simulink model "singlcontact_control_smc_lqr_mydimes_reaction"  (R2024a)
settings: Solver=VariableStepAuto  StartTime=0.0  StopTime=10  FixedStep=0.001  RelTol=1e-3
values from neighbouring files (symbols this model uses):
  ankle_servo_kd = 8    [robotParametersCtrl_mydiem_block_zmp.m]    (also in robotParametersCtrl_quad_modify_mydiem.m; robotParametersCtrl_quad_modify_mydiem_reaction.m)
  ankle_servo_ki = 4    [robotParametersCtrl_mydiem_block_zmp.m]    (also in robotParametersCtrl_quad_modify_mydiem.m; robotParametersCtrl_quad_modify_mydiem_reaction.m)
  ankle_servo_kp = 20    [robotParametersCtrl_mydiem_block_zmp.m]    (also in robotParametersCtrl_quad_modify_mydiem.m; robotParametersCtrl_quad_modify_mydiem_reaction.m)
  deriv_filter_coeff = 100    [robotParametersCtrl_mydiem_block_zmp.m]    (also in robotParametersCtrl_quad_modify_mydiem.m; robotParametersCtrl_quad_modify_mydiem_reaction.m)
  filter_coefficent_pid = 100    [robotParametersCtrl_mydiem_block_zmp.m]    (also in robotParametersCtrl_quad_modify_mydiem.m; robotParametersCtrl_quad_modify_mydiem_reaction.m)
  filter_coefficent_pids = 100    [robotParametersCtrl_quad_modify_mydiem_reaction.m]
  foot_z = 1.5    [robotParametersCtrl_mydiem_block_zmp.m]    (also in robotParametersCtrl_quad_modify_mydiem.m; robotParametersCtrl_quad_modify_mydiem_reaction.m)
  g = 9.81    [ABCDvalues_lqr_quad_mydime_reaction.m]    (also in robotParametersCtrl_mydiem_block_zmp.m = 9.80665; robotParametersCtrl_quad_modify_mydiem.m = 9.80665; robotParametersCtrl_quad_modify_mydiem_reaction.m = 9.80665)
  h = 32    [robotParametersCtrl_mydiem_block_zmp.m]    (also in robotParametersCtrl_quad_modify_mydiem.m; robotParametersCtrl_quad_modify_mydiem_reaction.m)
  height_plane = 0.025    [robotParametersCtrl_mydiem_block_zmp.m]    (also in robotParametersCtrl_quad_modify_mydiem.m; robotParametersCtrl_quad_modify_mydiem_reaction.m)
  hip_pitch_deriv = 20    [robotParametersCtrl_mydiem_block_zmp.m]    (also in robotParametersCtrl_quad_modify_mydiem.m = 200; robotParametersCtrl_quad_modify_mydiem_reaction.m = 200)
  hip_pitch_derivs = 200    [robotParametersCtrl_quad_modify_mydiem_reaction.m]
  hip_pitch_int = 0    [robotParametersCtrl_mydiem_block_zmp.m]    (also in robotParametersCtrl_quad_modify_mydiem.m = 150; robotParametersCtrl_quad_modify_mydiem_reaction.m = 150)
  hip_pitch_ints = 1500    [robotParametersCtrl_quad_modify_mydiem_reaction.m]
  hip_pitch_prop = 10    [robotParametersCtrl_mydiem_block_zmp.m]    (also in robotParametersCtrl_quad_modify_mydiem.m = 500; robotParametersCtrl_quad_modify_mydiem_reaction.m = 500)
  hip_pitch_props = 500    [robotParametersCtrl_quad_modify_mydiem_reaction.m]
  hip_roll_deriv = 28    [robotParametersCtrl_mydiem_block_zmp.m]    (also in robotParametersCtrl_quad_modify_mydiem.m = 280; robotParametersCtrl_quad_modify_mydiem_reaction.m = 280)
  hip_roll_derivs = 280    [robotParametersCtrl_quad_modify_mydiem_reaction.m]
  hip_roll_int = 0    [robotParametersCtrl_mydiem_block_zmp.m]    (also in robotParametersCtrl_quad_modify_mydiem.m = 180; robotParametersCtrl_quad_modify_mydiem_reaction.m = 180)
  hip_roll_ints = 180    [robotParametersCtrl_quad_modify_mydiem_reaction.m]
  hip_roll_prop = 10    [robotParametersCtrl_mydiem_block_zmp.m]    (also in robotParametersCtrl_quad_modify_mydiem.m = 300; robotParametersCtrl_quad_modify_mydiem_reaction.m = 300)
  hip_roll_props = 300    [robotParametersCtrl_quad_modify_mydiem_reaction.m]
  hip_servo_kd = 20    [robotParametersCtrl_mydiem_block_zmp.m]    (also in robotParametersCtrl_quad_modify_mydiem.m; robotParametersCtrl_quad_modify_mydiem_reaction.m)
  hip_servo_ki = 10    [robotParametersCtrl_mydiem_block_zmp.m]    (also in robotParametersCtrl_quad_modify_mydiem.m; robotParametersCtrl_quad_modify_mydiem_reaction.m)
  hip_servo_kp = 60    [robotParametersCtrl_mydiem_block_zmp.m]    (also in robotParametersCtrl_quad_modify_mydiem.m; robotParametersCtrl_quad_modify_mydiem_reaction.m)
  hip_smc_lamda = 85    [robotParametersCtrl_mydiem_block_zmp.m]    (also in robotParametersCtrl_quad_modify_mydiem.m; robotParametersCtrl_quad_modify_mydiem_reaction.m = 95)
  hip_smc_lamdas = 85    [robotParametersCtrl_quad_modify_mydiem_reaction.m]
  hip_smc_new = 25    [robotParametersCtrl_mydiem_block_zmp.m]    (also in robotParametersCtrl_quad_modify_mydiem.m; robotParametersCtrl_quad_modify_mydiem_reaction.m = 45)
  hip_smc_news = 25    [robotParametersCtrl_quad_modify_mydiem_reaction.m]
  init_angs_L = init_angs_R    [robotParametersCtrl_mydiem_block_zmp.m]    (also in robotParametersCtrl_quad_modify_mydiem.m; robotParametersCtrl_quad_modify_mydiem_reaction.m)
  init_angs_R = [0 -sum(init_angs) init_angs(2) 0 init_angs(1)]    [robotParametersCtrl_mydiem_block_zmp.m]    (also in robotParametersCtrl_quad_modify_mydiem.m; robotParametersCtrl_quad_modify_mydiem_reaction.m)
  init_height = h +                torso_z/2 + torso_offset_z + height_plane/2    (= 39.5125)    [robotParametersCtrl_mydiem_block_zmp.m]    (also in robotParametersCtrl_quad_modify_mydiem.m; robotParametersCtrl_quad_modify_mydiem_reaction.m)
  K = lqr(A, B, Q, R)    [ABCDvalues_lqr_quad_mydime_reaction.m]
  knee_pitch_deriv = 10    [robotParametersCtrl_mydiem_block_zmp.m]    (also in robotParametersCtrl_quad_modify_mydiem.m = 100; robotParametersCtrl_quad_modify_mydiem_reaction.m = 100)
  knee_pitch_derivs = 180    [robotParametersCtrl_quad_modify_mydiem_reaction.m]
  knee_pitch_int = 0    [robotParametersCtrl_mydiem_block_zmp.m]    (also in robotParametersCtrl_quad_modify_mydiem.m = 300; robotParametersCtrl_quad_modify_mydiem_reaction.m = 300)
  knee_pitch_ints = 7500    [robotParametersCtrl_quad_modify_mydiem_reaction.m]
  knee_pitch_prop = 10    [robotParametersCtrl_mydiem_block_zmp.m]    (also in robotParametersCtrl_quad_modify_mydiem.m = 400; robotParametersCtrl_quad_modify_mydiem_reaction.m = 400)
  knee_pitch_props = 1200    [robotParametersCtrl_quad_modify_mydiem_reaction.m]
  knee_servo_kd = 10    [robotParametersCtrl_mydiem_block_zmp.m]    (also in robotParametersCtrl_quad_modify_mydiem.m; robotParametersCtrl_quad_modify_mydiem_reaction.m)
  knee_servo_ki = 5    [robotParametersCtrl_mydiem_block_zmp.m]    (also in robotParametersCtrl_quad_modify_mydiem.m; robotParametersCtrl_quad_modify_mydiem_reaction.m)
  knee_servo_kp = 60    [robotParametersCtrl_mydiem_block_zmp.m]    (also in robotParametersCtrl_quad_modify_mydiem.m; robotParametersCtrl_quad_modify_mydiem_reaction.m)
  knee_smc_lamda = 140    [robotParametersCtrl_mydiem_block_zmp.m]    (also in robotParametersCtrl_quad_modify_mydiem.m; robotParametersCtrl_quad_modify_mydiem_reaction.m = 150)
  knee_smc_lamdas = 100    [robotParametersCtrl_quad_modify_mydiem_reaction.m]
  knee_smc_new = 80    [robotParametersCtrl_mydiem_block_zmp.m]    (also in robotParametersCtrl_quad_modify_mydiem.m; robotParametersCtrl_quad_modify_mydiem_reaction.m)
  knee_smc_news = 60    [robotParametersCtrl_quad_modify_mydiem_reaction.m]
  Kwalk = 0.6    [robotParametersCtrl_mydiem_block_zmp.m]    (also in robotParametersCtrl_quad_modify_mydiem.m; robotParametersCtrl_quad_modify_mydiem_reaction.m)
  l1 = 0.20    (= 0.2)    [ABCDvalues_lqr_quad_mydime_reaction.m]
  l2 = 0.20    (= 0.2)    [ABCDvalues_lqr_quad_mydime_reaction.m]
  lower_leg_length = 20    [robotParametersCtrl_mydiem_block_zmp.m]    (also in robotParametersCtrl_quad_modify_mydiem.m; robotParametersCtrl_quad_modify_mydiem_reaction.m)
  m1 = 0.45    [ABCDvalues_lqr_quad_mydime_reaction.m]
  m2 = 0.065    [ABCDvalues_lqr_quad_mydime_reaction.m]
  max_torque = 20    [robotParametersCtrl_mydiem_block_zmp.m]    (also in robotParametersCtrl_quad_modify_mydiem.m; robotParametersCtrl_quad_modify_mydiem_reaction.m)
  motion_time_constant = 0.01    [robotParametersCtrl_mydiem_block_zmp.m]    (also in robotParametersCtrl_quad_modify_mydiem.m; robotParametersCtrl_quad_modify_mydiem_reaction.m)
  plane_x = 25    [robotParametersCtrl_mydiem_block_zmp.m]    (also in robotParametersCtrl_quad_modify_mydiem.m; robotParametersCtrl_quad_modify_mydiem_reaction.m)
  plane_y = 3    [robotParametersCtrl_mydiem_block_zmp.m]    (also in robotParametersCtrl_quad_modify_mydiem.m; robotParametersCtrl_quad_modify_mydiem_reaction.m)
  stepHeight = 0.4    [ABCDvalues_lqr_quad_mydime_reaction.m]
  torso_offset_x = 17    [robotParametersCtrl_mydiem_block_zmp.m]    (also in robotParametersCtrl_quad_modify_mydiem.m; robotParametersCtrl_quad_modify_mydiem_reaction.m)
  torso_offset_x1 = -17    [robotParametersCtrl_mydiem_block_zmp.m]    (also in robotParametersCtrl_quad_modify_mydiem.m; robotParametersCtrl_quad_modify_mydiem_reaction.m)
  torso_offset_z = 0    [robotParametersCtrl_mydiem_block_zmp.m]    (also in robotParametersCtrl_quad_modify_mydiem.m; robotParametersCtrl_quad_modify_mydiem_reaction.m)
  torso_x = 40    [robotParametersCtrl_mydiem_block_zmp.m]    (also in robotParametersCtrl_quad_modify_mydiem.m; robotParametersCtrl_quad_modify_mydiem_reaction.m)
  torso_y = 20    [robotParametersCtrl_mydiem_block_zmp.m]    (also in robotParametersCtrl_quad_modify_mydiem.m; robotParametersCtrl_quad_modify_mydiem_reaction.m)
  torso_z = 15    [robotParametersCtrl_mydiem_block_zmp.m]    (also in robotParametersCtrl_quad_modify_mydiem.m; robotParametersCtrl_quad_modify_mydiem_reaction.m)
  Ts = 0.05    [ABCDvalues_lqr_quad_mydime_reaction.m]
  TsCtrl = 0.05    [robotParametersCtrl_mydiem_block_zmp.m]    (also in robotParametersCtrl_quad_modify_mydiem.m; robotParametersCtrl_quad_modify_mydiem_reaction.m)
  tWalk = 0.3    [robotParametersCtrl_mydiem_block_zmp.m]    (also in robotParametersCtrl_quad_modify_mydiem.m; robotParametersCtrl_quad_modify_mydiem_reaction.m)
  upper_leg_length = 20    [robotParametersCtrl_mydiem_block_zmp.m]    (also in robotParametersCtrl_quad_modify_mydiem.m; robotParametersCtrl_quad_modify_mydiem_reaction.m)
undefined symbols (not defined in the file or in its folder): X, Y, Z
libraries: simulink_extras x256, slpidlib x128, sm_lib x71, simulink x43, nesl_utility x35, walkingRobotUtils x21, dspsrcs4 x18, dspobslib x8
(part 28 of 33)

== system singlcontact_control_smc_lqr_mydimes_reaction/Walking Robot/smc+smcr+neuro1+reaction2/SMC Controllers FR2/SMC ==
  In1 : Inport
  In2 : Inport  Port=2
  T1_neuro : Inport  Port=3
  T2_neuro : Inport  Port=4
  Add : Sum
  Add1 : Sum
  Edot : Derivative
  Edot1 : Derivative
  Gain : Gain  Gain=-0.9
  Gain1 : Gain  Gain=-0.9
  Mux : Mux  Inputs=2
  New : Gain  Gain=25
  New1 : Gain  Gain=25
  Product : Product
  Product2 : Product
  S : Sum
  S1 : Sum
  Scope : Scope  NumInputPorts=2
  Scope{2..5} (4 alike) : Scope
  Sum : Sum  Inputs=++++
  Sum1 : Sum  Inputs=++++
  Tanh : Trigonometry  Operator=tanh
  Tanh1 : Trigonometry  Operator=tanh
  lamda : Constant  Value=50
  lamda1 : Constant  Value=50
  Out1 : Outport
  tag scope: edotBR1=global, edotBR2=global, lamdaBR1=global, lamdaBR2=global
  wires:
  S1/1 -> Tanh/1
  Edot/1 -> [edotBR1], S/1
  Product/1 -> S/2
  lamda1/1 -> [lamdaBR2], Product2/1
  In2/1 -> Product2/2, Edot1/1
  New1/1 -> Add1/1, Sum1/1
  Product2/1 -> S1/2
  In1/1 -> Edot/1, Product/2
  Edot1/1 -> S1/1, [edotBR2]
  Tanh1/1 -> New/1
  lamda/1 -> [lamdaBR1], Product/1
  Tanh/1 -> New1/1
  New/1 -> Sum/1, Add/1, Scope/1
  [TT1BR] -> Scope/2, Add/2, Sum/2
  [TT2BR] -> Add1/2, Sum1/2
  Mux/1 -> Out1/1
  Sum/1 -> Scope3/1, Scope5/1, Mux/1
  Sum1/1 -> Scope4/1, Mux/2, Scope2/1
  T1_neuro/1 -> ?
  T2_neuro/1 -> ?
  S/1 -> Tanh1/1
  Add/1 -> Gain/1
  Gain/1 -> ?
  Gain1/1 -> ?
  Add1/1 -> Gain1/1

== system singlcontact_control_smc_lqr_mydimes_reaction/Walking Robot/smc+smcr+neuro1+reaction2/SMC Controllers FR3/Equivalent control ==
  theta2 : Inport
  theta1 : Inport  Port=2
  theta2ddot : Inport  Port=3
  theta1dot : Inport  Port=4
  theta2dot : Inport  Port=5
  theta1ddot : Inport  Port=6
  theta3 : Inport  Port=7
  theta4 : Inport  Port=8
  theta1dot1 : Inport  Port=9
  Constant : Constant  Value=0
  Constant1 : Constant  Value=0
  SMC equivalent T1 : Subsystem
  SMC equivalent T2 : Subsystem
  Scope : Scope  NumInputPorts=2
  tag scope: TT1BL=global, TT2BL=global
  wires:
  theta1dot1/1 -> SMC equivalent T2/5(theta1dot)
  theta2dot/1 -> SMC equivalent T1/5(theta2dot)
  theta1ddot/1 -> SMC equivalent T2/1(theta1ddot)
  theta4/1 -> SMC equivalent T2/3(theta1)
  theta1/1 -> SMC equivalent T1/2(theta1)
  theta3/1 -> SMC equivalent T2/2(theta2)
  Constant/1 -> SMC equivalent T1/6(theta1ddot)
  theta1dot/1 -> SMC equivalent T1/4(theta1dot)
  theta2ddot/1 -> SMC equivalent T1/3(theta2ddot)
  Constant1/1 -> SMC equivalent T2/4(theta2ddot)
  SMC equivalent T1/1(T1) -> [TT1BL], Scope/2
  theta2/1 -> SMC equivalent T1/1(theta2)
  SMC equivalent T2/1(T2) -> [TT2BL], Scope/1

== system singlcontact_control_smc_lqr_mydimes_reaction/Walking Robot/smc+smcr+neuro1+reaction2/SMC Controllers FR3/SMC ==
  In1 : Inport
  In2 : Inport  Port=2
  T1_neuro : Inport  Port=3
  T2_neuro : Inport  Port=4
  Add : Sum
  Add1 : Sum
  Edot : Derivative
  Edot1 : Derivative
  Gain : Gain  Gain=-0.9
  Gain1 : Gain  Gain=-0.9
  Mux : Mux  Inputs=2
  New : Gain  Gain=25
  New1 : Gain  Gain=25
  Product : Product
  Product2 : Product
  S : Sum
  S1 : Sum
  Scope : Scope  NumInputPorts=2
  Scope{2..5} (4 alike) : Scope
  Sum : Sum  Inputs=++++
  Sum1 : Sum  Inputs=++++
  Tanh : Trigonometry  Operator=tanh
  Tanh1 : Trigonometry  Operator=tanh
  lamda : Constant  Value=50
  lamda1 : Constant  Value=50
  Out1 : Outport
  tag scope: edotBL1=global, edotBL2=global, lamdaBL1=global, lamdaBL2=global
  wires:
  Add1/1 -> Gain1/1
  Gain1/1 -> ?
  Gain/1 -> ?
  Add/1 -> Gain/1
  S/1 -> Tanh1/1
  T2_neuro/1 -> ?
  T1_neuro/1 -> ?
  Sum1/1 -> Scope2/1, Mux/2, Scope4/1
  Sum/1 -> Mux/1, Scope5/1, Scope3/1
  Mux/1 -> Out1/1
  [TT2BL] -> Sum1/2, Add1/2
  [TT1BL] -> Sum/2, Add/2, Scope/2
  New/1 -> Scope/1, Add/1, Sum/1
  Tanh/1 -> New1/1
  lamda/1 -> Product/1, [lamdaBL1]
  Tanh1/1 -> New/1
  Edot1/1 -> [edotBL2], S1/1
  In1/1 -> Product/2, Edot/1
  Product2/1 -> S1/2
  New1/1 -> Sum1/1, Add1/1
  In2/1 -> Edot1/1, Product2/2
  lamda1/1 -> Product2/1, [lamdaBL2]
  Product/1 -> S/2
  Edot/1 -> S/1, [edotBL1]
  S1/1 -> Tanh/1

== system singlcontact_control_smc_lqr_mydimes_reaction/Walking Robot/smc+smcr+neuro1+reaction2/SMC Controllers FR4/Equivalent control ==
  theta2 : Inport
  theta1 : Inport  Port=2
  theta2ddot : Inport  Port=3
  theta1dot : Inport  Port=4
  theta2dot : Inport  Port=5
  theta1ddot : Inport  Port=6
  theta3 : Inport  Port=7
  theta4 : Inport  Port=8
  theta1dot1 : Inport  Port=9
  Constant : Constant  Value=0
  Constant1 : Constant  Value=0
  SMC equivalent T1 : Subsystem
  SMC equivalent T2 : Subsystem
  Scope : Scope  NumInputPorts=2
  tag scope: TT1FRss=global, TT2FRss=global
  wires:
  SMC equivalent T2/1(T2) -> Scope/1, [TT2FRss]
  theta2/1 -> SMC equivalent T1/1(theta2)
  SMC equivalent T1/1(T1) -> Scope/2, [TT1FRss]
  Constant1/1 -> SMC equivalent T2/4(theta2ddot)
  theta2ddot/1 -> SMC equivalent T1/3(theta2ddot)
  theta1dot/1 -> SMC equivalent T1/4(theta1dot)
  Constant/1 -> SMC equivalent T1/6(theta1ddot)
  theta3/1 -> SMC equivalent T2/2(theta2)
  theta1/1 -> SMC equivalent T1/2(theta1)
  theta4/1 -> SMC equivalent T2/3(theta1)
  theta1ddot/1 -> SMC equivalent T2/1(theta1ddot)
  theta2dot/1 -> SMC equivalent T1/5(theta2dot)
  theta1dot1/1 -> SMC equivalent T2/5(theta1dot)

== system singlcontact_control_smc_lqr_mydimes_reaction/Walking Robot/smc+smcr+neuro1+reaction2/SMC Controllers FR4/SMC ==
  In1 : Inport
  In2 : Inport  Port=2
  T1_neuro : Inport  Port=3
  T2_neuro : Inport  Port=4
  Edot : Derivative
  Edot1 : Derivative
  Gain : Gain  Gain=-0.5
  Gain1 : Gain  Gain=-0.5
  Mux : Mux  Inputs=2
  New : Gain  Gain=knee_smc_new
  New1 : Gain  Gain=hip_smc_new
  Product : Product
  Product2 : Product
  Random Source : dspsrcs4/Random Source  SrcType=Uniform  NormMethod=Ziggurat  CltLength=12  MinVal=0  MaxVal=1  MeanVal=0  VarVal=1  RepMode=Not repeatable  rawSeed=1  IsInherit=off  SampMode=Discrete  SampTime=0.05  SampFrame=1  DataType=Double  OutComplex=Real  OutputFrames=off
  S : Sum
  S1 : Sum
  Scope{,1..6} (7 alike) : Scope
  Sum : Sum  Inputs=+++++
  Sum1 : Sum  Inputs=+++++
  Tanh : Trigonometry  Operator=tanh
  Tanh1 : Trigonometry  Operator=tanh
  lamda : Constant  Value=knee_smc_lamda
  lamda1 : Constant  Value=hip_smc_lamda
  Out1 : Outport
  tag scope: edotFR1s=global, edotFR2s=global, lamdaFR1s=global, lamdaFR2s=global, slFR1s=global, slFR2s=global
  wires:
  S1/1 -> [slFR2s], Tanh/1
  Edot/1 -> [edotFR1s], S/1
  Product/1 -> S/2
  lamda1/1 -> [lamdaFR2s], Product2/1
  In2/1 -> Product2/2, Edot1/1
  Product2/1 -> S1/2
  In1/1 -> Edot/1, Product/2
  Edot1/1 -> S1/1, [edotFR2s]
  Tanh1/1 -> New/1
  lamda/1 -> [lamdaFR1s], Product/1
  Tanh/1 -> New1/1
  [TT1FRs] -> Sum/2
  [TT2FRs] -> Sum1/2
  Mux/1 -> Out1/1
  Sum/1 -> Scope3/1, Scope5/1, Mux/1
  Sum1/1 -> Scope4/1, Mux/2, Scope2/1
  T1_neuro/1 -> ?
  T2_neuro/1 -> ?
  S/1 -> [slFR1s], Tanh1/1
  New/1 -> Gain/1, Sum/1
  Gain/1 -> ?
  Gain1/1 -> ?
  New1/1 -> Gain1/1, Sum1/1
  Random Source/1 -> ?
  ? -> Scope/1

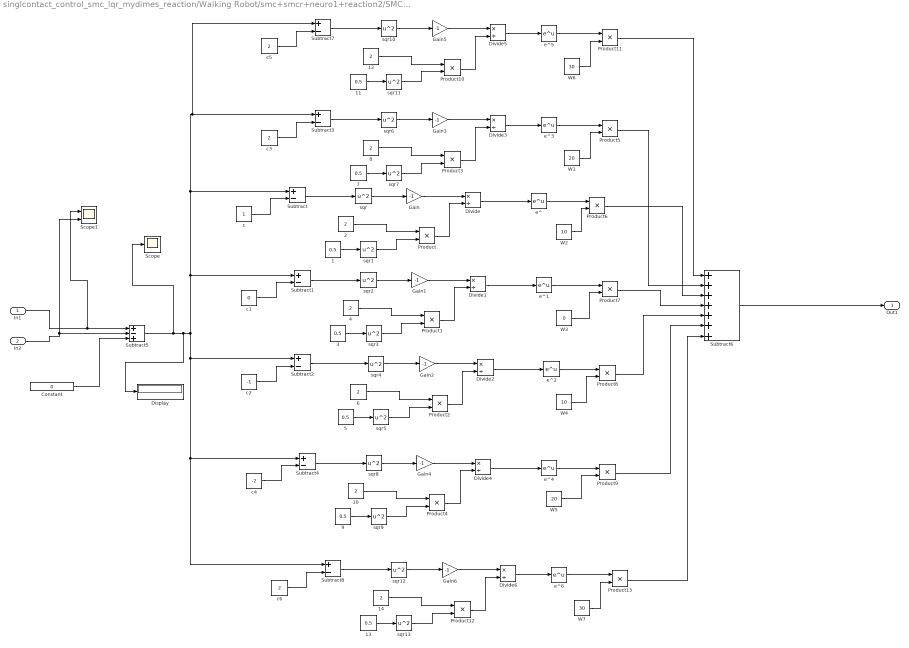
== system singlcontact_control_smc_lqr_mydimes_reaction/Walking Robot/smc+smcr+neuro1+reaction2/SMC Controllers FR4/Subsystem ==
  In1 : Inport
  In2 : Inport  Port=2
  {1,3,5,7,9,11,13} (7 alike) : Constant  Value=0.5
  {2,4,6,8,10,12,14} (7 alike) : Constant  Value=2
  Constant : Constant  Value=0
  Display : Display
  Divide{,1..6} (7 alike) : Product  Inputs=*/
  Gain{,1..6} (7 alike) : Gain  Gain=-1
  Product{,1..13} (14 alike) : Product
  Scope : Scope
  Scope1 : Scope  NumInputPorts=2
  Subtract{,1..4,7..8} (7 alike) : Sum  Inputs=+-
  Subtract5 : Sum  Inputs=+-+
  Subtract6 : Sum  Inputs=+++++++
  W1 : Constant  Value=20
  W2 : Constant  Value=10
  W3 : Constant  Value=0
  W4 : Constant  Value=10
  W5 : Constant  Value=20
  W6 : Constant  Value=30
  W7 : Constant  Value=30
  c : Constant
  c1 : Constant  Value=0
  c2 : Constant  Value=-1
  c3 : Constant  Value=2
  c4 : Constant  Value=-2
  c5 : Constant  Value=2
  c6 : Constant  Value=2
  e^{,1..6} (7 alike) : Math
  sqr{,1..13} (14 alike) : Math  Operator=square
  Out1 : Outport
  wires:
  c/1 -> Subtract/2
  sqr9/1 -> Product4/2
  Product1/1 -> Divide1/2
  sqr/1 -> Gain/1
  Product/1 -> Divide/2
  sqr2/1 -> Gain1/1
  sqr1/1 -> Product/2
  In2/1 -> Subtract5/2, Scope1/2
  Gain3/1 -> Divide3/1
  Divide1/1 -> e^1/1
  Subtract4/1 -> sqr8/1
  Gain/1 -> Divide/1
  Product2/1 -> Divide2/2
  Product6/1 -> Subtract6/3
  Gain1/1 -> Divide1/1
  W3/1 -> Product7/2
  W2/1 -> Product6/2
  Product3/1 -> Divide3/2
  e^/1 -> Product6/1
  Subtract3/1 -> sqr6/1
  c4/1 -> Subtract4/2
  Product9/1 -> Subtract6/6
  e^1/1 -> Product7/1
  Subtract1/1 -> sqr2/1
  c1/1 -> Subtract1/2
  Subtract/1 -> sqr/1
  7/1 -> sqr7/1
  W5/1 -> Product9/2
  Divide4/1 -> e^4/1
  Product5/1 -> Subtract6/2
  2/1 -> Product/1
  1/1 -> sqr1/1
  sqr8/1 -> Gain4/1
  sqr5/1 -> Product2/2
  e^4/1 -> Product9/1
  c3/1 -> Subtract3/2
  sqr4/1 -> Gain2/1
  W1/1 -> Product5/2
  In1/1 -> Scope1/1, Subtract5/1
  Gain4/1 -> Divide4/1
  Gain2/1 -> Divide2/1
  4/1 -> Product1/1
  3/1 -> sqr3/1
  5/1 -> sqr5/1
  Divide/1 -> e^/1
  sqr7/1 -> Product3/2
  8/1 -> Product3/1
  Subtract6/1 -> Out1/1
  Subtract2/1 -> sqr4/1
  Divide2/1 -> e^2/1
  e^2/1 -> Product8/1
  sqr3/1 -> Product1/2
  6/1 -> Product2/1
  sqr6/1 -> Gain3/1
  e^3/1 -> Product5/1
  10/1 -> Product4/1
  Product4/1 -> Divide4/2
  c2/1 -> Subtract2/2
  W4/1 -> Product8/2
  Product7/1 -> Subtract6/4
  Product8/1 -> Subtract6/5
  9/1 -> sqr9/1
  Divide3/1 -> e^3/1
  Constant/1 -> Subtract5/3
  Divide5/1 -> e^5/1
  12/1 -> Product10/1
  sqr10/1 -> Gain5/1
  11/1 -> sqr11/1
  c5/1 -> Subtract7/2
  Gain5/1 -> Divide5/1
  e^5/1 -> Product11/1
  Product11/1 -> Subtract6/1
  Subtract7/1 -> sqr10/1
  Product10/1 -> Divide5/2
  W6/1 -> Product11/2
  sqr11/1 -> Product10/2
  Divide6/1 -> e^6/1
  14/1 -> Product12/1
  Subtract5/1 -> Scope/1, Display/1, Subtract1/1, Subtract/1, Subtract7/1, Subtract3/1, Subtract8/1, Subtract4/1, Subtract2/1
  sqr12/1 -> Gain6/1
  13/1 -> sqr13/1
  c6/1 -> Subtract8/2
  Gain6/1 -> Divide6/1
  e^6/1 -> Product13/1
  Subtract8/1 -> sqr12/1
  Product12/1 -> Divide6/2
  W7/1 -> Product13/2
  sqr13/1 -> Product12/2
  Product13/1 -> Subtract6/7

== system singlcontact_control_smc_lqr_mydimes_reaction/Walking Robot/smc+smcr+neuro1+reaction2/SMC Controllers FR4/Subsystem1 ==
  In1 : Inport
  In2 : Inport  Port=2
  {1,3,5,7,9} (5 alike) : Constant  Value=0.5
  {2,4,6,8,10} (5 alike) : Constant  Value=2
  Constant : Constant  Value=0
  Display : Display
  Divide{,1..4} (5 alike) : Product  Inputs=*/
  Gain{,1..4} (5 alike) : Gain  Gain=-1
  Product{,1..9} (10 alike) : Product
  Scope : Scope
  Scope1 : Scope  NumInputPorts=2
  Subtract{,1..4} (5 alike) : Sum  Inputs=+-
  Subtract5 : Sum  Inputs=+-+
  Subtract6 : Sum  Inputs=+++++
  W1 : Constant  Value=20
  W2 : Constant  Value=10
  W3 : Constant  Value=0
  W4 : Constant  Value=10
  W5 : Constant  Value=20
  c : Constant
  c1 : Constant  Value=0
  c2 : Constant  Value=-1
  c3 : Constant  Value=2
  c4 : Constant  Value=-2
  e^{,1..4} (5 alike) : Math
  sqr{,1..9} (10 alike) : Math  Operator=square
  Out1 : Outport
  wires:
  Constant/1 -> Subtract5/3
  Divide3/1 -> e^3/1
  9/1 -> sqr9/1
  Product8/1 -> Subtract6/4
  Product7/1 -> Subtract6/3
  W4/1 -> Product8/2
  c2/1 -> Subtract2/2
  Product4/1 -> Divide4/2
  10/1 -> Product4/1
  e^3/1 -> Product5/1
  sqr6/1 -> Gain3/1
  6/1 -> Product2/1
  sqr3/1 -> Product1/2
  e^2/1 -> Product8/1
  Divide2/1 -> e^2/1
  Subtract2/1 -> sqr4/1
  Subtract6/1 -> Out1/1
  8/1 -> Product3/1
  sqr7/1 -> Product3/2
  Divide/1 -> e^/1
  5/1 -> sqr5/1
  3/1 -> sqr3/1
  4/1 -> Product1/1
  Gain2/1 -> Divide2/1
  Gain4/1 -> Divide4/1
  In1/1 -> Subtract5/1, Scope1/1
  W1/1 -> Product5/2
  sqr4/1 -> Gain2/1
  c3/1 -> Subtract3/2
  e^4/1 -> Product9/1
  sqr5/1 -> Product2/2
  sqr8/1 -> Gain4/1
  1/1 -> sqr1/1
  2/1 -> Product/1
  Product5/1 -> Subtract6/1
  Divide4/1 -> e^4/1
  W5/1 -> Product9/2
  7/1 -> sqr7/1
  Subtract/1 -> sqr/1
  Subtract5/1 -> Subtract2/1, Subtract4/1, Subtract3/1, Subtract/1, Subtract1/1, Display/1, Scope/1
  c1/1 -> Subtract1/2
  Subtract1/1 -> sqr2/1
  e^1/1 -> Product7/1
  Product9/1 -> Subtract6/5
  c4/1 -> Subtract4/2
  Subtract3/1 -> sqr6/1
  e^/1 -> Product6/1
  Product3/1 -> Divide3/2
  W2/1 -> Product6/2
  W3/1 -> Product7/2
  Gain1/1 -> Divide1/1
  Product6/1 -> Subtract6/2
  Product2/1 -> Divide2/2
  Gain/1 -> Divide/1
  Subtract4/1 -> sqr8/1
  Divide1/1 -> e^1/1
  Gain3/1 -> Divide3/1
  In2/1 -> Scope1/2, Subtract5/2
  sqr1/1 -> Product/2
  sqr2/1 -> Gain1/1
  Product/1 -> Divide/2
  sqr/1 -> Gain/1
  Product1/1 -> Divide1/2
  sqr9/1 -> Product4/2
  c/1 -> Subtract/2

== system singlcontact_control_smc_lqr_mydimes_reaction/Walking Robot/Lqr+Lqr+reaction/LQR2 Controllers BL/Subsystem2/length from ground ==
  In1 : Inport
  In2 : Inport  Port=2
  Gain1 : Gain  Gain=l1
  Gain3 : Gain  Gain=l1
  Gain4 : Gain  Gain=l2
  Sin : Trigonometry
  Sin1 : Trigonometry
  Sin3 : Trigonometry
  Sum : Sum  Inputs=|++
  Sum2 : Sum  Inputs=|++
  Output : Outport
  Outport : Outport  Port=2
  wires:
  In2/1 -> Sum2/2
  Sin3/1 -> Gain4/1
  Gain1/1 -> Output/1
  Sin1/1 -> Gain3/1
  Sum2/1 -> Sin3/1
  Gain3/1 -> Sum/1
  Gain4/1 -> Sum/2
  Sum/1 -> Outport/1
  Sin/1 -> Gain1/1
  In1/1 -> Sin1/1, Sum2/1, Sin/1

== system singlcontact_control_smc_lqr_mydimes_reaction/Walking Robot/Lqr+Lqr+reaction/LQR2 Controllers BR/Subsystem2/length from ground ==
  In1 : Inport
  In2 : Inport  Port=2
  Gain1 : Gain  Gain=l1
  Gain3 : Gain  Gain=l1
  Gain4 : Gain  Gain=l2
  Sin : Trigonometry
  Sin1 : Trigonometry
  Sin3 : Trigonometry
  Sum : Sum  Inputs=|++
  Sum2 : Sum  Inputs=|++
  Output : Outport
  Outport : Outport  Port=2
  wires:
  In1/1 -> Sin/1, Sum2/1, Sin1/1
  Sin/1 -> Gain1/1
  Gain4/1 -> Sum/2
  Gain3/1 -> Sum/1
  Sum2/1 -> Sin3/1
  Sin1/1 -> Gain3/1
  Sin3/1 -> Gain4/1
  In2/1 -> Sum2/2
  Sum/1 -> Outport/1
  Gain1/1 -> Output/1

== system singlcontact_control_smc_lqr_mydimes_reaction/Walking Robot/Lqr+Lqr+reaction/LQR2 Controllers FL/Subsystem2/length from ground ==
  In1 : Inport
  In2 : Inport  Port=2
  Gain1 : Gain  Gain=l1
  Gain3 : Gain  Gain=l1
  Gain4 : Gain  Gain=l2
  Sin : Trigonometry
  Sin1 : Trigonometry
  Sin3 : Trigonometry
  Sum : Sum  Inputs=|++
  Sum2 : Sum  Inputs=|++
  Output : Outport
  Outport : Outport  Port=2
  wires:
  In2/1 -> Sum2/2
  Sin3/1 -> Gain4/1
  Sin1/1 -> Gain3/1
  Sum2/1 -> Sin3/1
  Gain3/1 -> Sum/1
  Gain4/1 -> Sum/2
  Sin/1 -> Gain1/1
  In1/1 -> Sin1/1, Sum2/1, Sin/1
  Gain1/1 -> Output/1
  Sum/1 -> Outport/1

== system singlcontact_control_smc_lqr_mydimes_reaction/Walking Robot/Lqr+Lqr+reaction/LQR2 Controllers FR/Subsystem2/length from ground ==
  In1 : Inport
  In2 : Inport  Port=2
  Gain1 : Gain  Gain=l1
  Gain3 : Gain  Gain=l1
  Gain4 : Gain  Gain=l2
  Sin : Trigonometry
  Sin1 : Trigonometry
  Sin3 : Trigonometry
  Sum : Sum  Inputs=|++
  Sum2 : Sum  Inputs=|++
  Output : Outport
  Outport : Outport  Port=2
  wires:
  In1/1 -> Sin/1, Sum2/1, Sin1/1
  Sin/1 -> Gain1/1
  Gain4/1 -> Sum/2
  Gain3/1 -> Sum/1
  Sum2/1 -> Sin3/1
  Sin1/1 -> Gain3/1
  Sin3/1 -> Gain4/1
  In2/1 -> Sum2/2
  Gain1/1 -> Output/1
  Sum/1 -> Outport/1

== system singlcontact_control_smc_lqr_mydimes_reaction/Walking Robot/Lqr+Lqr+reaction/SMC Controllers FR1/Equivalent control/SMC equivalent T1 ==
  theta2 : Inport
  theta1 : Inport  Port=2
  theta2ddot : Inport  Port=3
  theta1dot : Inport  Port=4
  theta2dot : Inport  Port=5
  theta1ddot : Inport  Port=6
  Add{1..4} (4 alike) : Sum
  Add5 : Sum  Inputs=+--+++
  Add6 : Sum  Inputs=++++
  Constant : Constant  Value=0.3
  Constant10 : Constant  Value=m2*l1^2
  Constant11 : Constant  Value=0.3*m1*l1^2
  Constant12 : Constant  Value=m2*l1*l2
  Constant2 : Constant  Value=0.5
  Constant3 : Constant
  Constant4 : Constant  Value=0.5
  Constant5 : Constant
  Constant6 : Constant  Value=g*l1
  Constant7 : Constant  Value=0.5
  Constant9 : Constant  Value=0.3*m2*l2^2
  Cos : Trigonometry  Operator=cos
  Cos1 : Trigonometry  Operator=cos
  Gain1 : Gain  Gain=m2*l2^2
  Gain2 : Gain  Gain=m2*l2*l1
  Gain4 : Gain  Gain=m2*l2*l1
  Gain6 : Gain  Gain=m1
  Gain7 : Gain  Gain=m2
  Gain8 : Gain  Gain=m2*g*l2
  Product{1..3,7..9} (6 alike) : Product
  Product4 : Product  Inputs=4
  Product5 : Product  Inputs=3
  Product6 : Product  Inputs=3
  Sin : Trigonometry
  Sin1 : Trigonometry
  Sin2 : Trigonometry
  Square1 : Math  Operator=square
  T1 : Outport
  wires:
  Add2/1 -> Product1/1
  Product9/1 -> Add2/2
  [lamdaFL1] -> Product9/1
  [edotFL1] -> Product9/2
  Add5/1 -> T1/1
  Product1/1 -> Add5/6
  theta1ddot/1 -> Add2/1
  Add6/1 -> Product1/2
  Product8/1 -> Add6/1
  Constant11/1 -> Add6/2
  Constant10/1 -> Add6/4
  Constant9/1 -> Add6/3
  Cos1/1 -> Product8/1
  Constant12/1 -> Product8/2  "X_dd"
  theta2/1 -> Cos/1, Sin/1, Add4/1, Cos1/1
  Product7/1 -> Add5/5
  Product6/1 -> Add5/4
  Product5/1 -> Add5/3
  Product4/1 -> Add5/2
  Product3/1 -> Add5/1
  Sin2/1 -> Product7/2
  Gain8/1 -> Product7/1
  Add4/1 -> Sin2/1
  Constant7/1 -> Gain8/1
  Constant6/1 -> Product6/3
  Sin1/1 -> Product6/2
  Add3/1 -> Product6/1
  theta1/1 -> Sin1/1, Add4/2
  Gain6/1 -> Add3/1
  Gain7/1 -> Add3/2
  Constant5/1 -> Gain7/1
  Constant4/1 -> Gain6/1
  Square1/1 -> Product5/3
  Constant3/1 -> Gain4/1
  Gain4/1 -> Product4/1
  Sin/1 -> Product5/2, Product4/2
  theta2dot/1 -> Square1/1, Product4/4
  theta1dot/1 -> Product4/3
  Add1/1 -> Product3/2
  theta2ddot/1 -> Product3/1
  Product2/1 -> Add1/2
  Gain1/1 -> Add1/1
  Gain2/1 -> Product5/1, Product2/1
  Cos/1 -> Product2/2
  Constant2/1 -> Gain2/1
  Constant/1 -> Gain1/1

== system singlcontact_control_smc_lqr_mydimes_reaction/Walking Robot/Lqr+Lqr+reaction/SMC Controllers FR1/Equivalent control/SMC equivalent T2 ==
  theta1ddot : Inport
  theta2 : Inport  Port=2
  theta1 : Inport  Port=3
  theta2ddot : Inport  Port=4
  theta1dot : Inport  Port=5
  Add1 : Sum
  Add2 : Sum
  Add4 : Sum
  Add5 : Sum  Inputs=++++
  Constant : Constant  Value=0.5
  Constant1 : Constant  Value=0.3
  Constant2 : Constant  Value=0.5
  Constant3 : Constant
  Gain10 : Gain  Gain=m2*l2^2
  Gain11 : Gain  Gain=m2*l2
  Gain12 : Gain  Gain=g
  Gain13 : Gain  Gain=(1/3)*(m2*(l2^2))
  Gain5 : Gain  Gain=m2*l1*l2
  Product{1..4,7} (5 alike) : Product
  Product6 : Product  Inputs=3
  Sin : Trigonometry
  Square3 : Math  Operator=square
  Trigonometric Function3 : Trigonometry  Operator=cos
  Trigonometric Function4 : Trigonometry
  T2 : Outport
  wires:
  Product2/1 -> Add5/4
  Gain13/1 -> Product2/1
  Add1/1 -> Product2/2
  Constant3/1 -> Gain13/1
  theta2ddot/1 -> Add1/2
  [edotFL2] -> Product1/1
  [lamdaFL2] -> Product1/2
  Product1/1 -> Add1/1
  Add5/1 -> T2/1
  Product7/1 -> Add5/3
  Product6/1 -> Add5/2
  Product4/1 -> Add5/1
  Add4/1 -> Sin/1
  Sin/1 -> Product7/2
  theta1/1 -> Add4/1
  Gain12/1 -> Product7/1
  Gain11/1 -> Gain12/1
  Constant2/1 -> Gain11/1
  Square3/1 -> Product6/3
  theta1dot/1 -> Square3/1
  Trigonometric Function4/1 -> Product6/2
  Constant1/1 -> Gain10/1
  Constant/1 -> Gain5/1
  theta1ddot/1 -> Product4/1
  Add2/1 -> Product4/2
  Gain10/1 -> Add2/2
  Product3/1 -> Add2/1
  Gain5/1 -> Product6/1, Product3/2
  Trigonometric Function3/1 -> Product3/1
  theta2/1 -> Trigonometric Function4/1, Add4/2, Trigonometric Function3/1

== system singlcontact_control_smc_lqr_mydimes_reaction/Walking Robot/Lqr+Lqr+reaction/SMC Controllers FR2/Equivalent control/SMC equivalent T1 ==
  theta2 : Inport
  theta1 : Inport  Port=2
  theta2ddot : Inport  Port=3
  theta1dot : Inport  Port=4
  theta2dot : Inport  Port=5
  theta1ddot : Inport  Port=6
  Add{1..4} (4 alike) : Sum
  Add5 : Sum  Inputs=+--+++
  Add6 : Sum  Inputs=++++
  Constant : Constant  Value=0.3
  Constant10 : Constant  Value=m2*l1^2
  Constant11 : Constant  Value=0.3*m1*l1^2
  Constant12 : Constant  Value=m2*l1*l2
  Constant2 : Constant  Value=0.5
  Constant3 : Constant
  Constant4 : Constant  Value=0.5
  Constant5 : Constant
  Constant6 : Constant  Value=g*l1
  Constant7 : Constant  Value=0.5
  Constant9 : Constant  Value=0.3*m2*l2^2
  Cos : Trigonometry  Operator=cos
  Cos1 : Trigonometry  Operator=cos
  Gain1 : Gain  Gain=m2*l2^2
  Gain2 : Gain  Gain=m2*l2*l1
  Gain4 : Gain  Gain=m2*l2*l1
  Gain6 : Gain  Gain=m1
  Gain7 : Gain  Gain=m2
  Gain8 : Gain  Gain=m2*g*l2
  Product{1..3,7..9} (6 alike) : Product
  Product4 : Product  Inputs=4
  Product5 : Product  Inputs=3
  Product6 : Product  Inputs=3
  Sin : Trigonometry
  Sin1 : Trigonometry
  Sin2 : Trigonometry
  Square1 : Math  Operator=square
  T1 : Outport
  wires:
  Constant/1 -> Gain1/1
  Constant2/1 -> Gain2/1
  Cos/1 -> Product2/2
  Gain2/1 -> Product2/1, Product5/1
  Gain1/1 -> Add1/1
  Product2/1 -> Add1/2
  theta2ddot/1 -> Product3/1
  Add1/1 -> Product3/2
  theta1dot/1 -> Product4/3
  theta2dot/1 -> Product4/4, Square1/1
  Sin/1 -> Product4/2, Product5/2
  Gain4/1 -> Product4/1
  Constant3/1 -> Gain4/1
  Square1/1 -> Product5/3
  Constant4/1 -> Gain6/1
  Constant5/1 -> Gain7/1
  Gain7/1 -> Add3/2
  Gain6/1 -> Add3/1
  theta1/1 -> Add4/2, Sin1/1
  Add3/1 -> Product6/1
  Sin1/1 -> Product6/2
  Constant6/1 -> Product6/3
  Constant7/1 -> Gain8/1
  Add4/1 -> Sin2/1
  Gain8/1 -> Product7/1
  Sin2/1 -> Product7/2
  Product3/1 -> Add5/1
  Product4/1 -> Add5/2
  Product5/1 -> Add5/3
  Product6/1 -> Add5/4
  Product7/1 -> Add5/5
  theta2/1 -> Cos1/1, Add4/1, Sin/1, Cos/1
  Constant12/1 -> Product8/2  "X_dd"
  Cos1/1 -> Product8/1
  Constant9/1 -> Add6/3
  Constant10/1 -> Add6/4
  Constant11/1 -> Add6/2
  Product8/1 -> Add6/1
  Add6/1 -> Product1/2
  theta1ddot/1 -> Add2/1
  Product1/1 -> Add5/6
  Add5/1 -> T1/1
  [edotBR1] -> Product9/2
  [lamdaBR1] -> Product9/1
  Product9/1 -> Add2/2
  Add2/1 -> Product1/1

== system singlcontact_control_smc_lqr_mydimes_reaction/Walking Robot/Lqr+Lqr+reaction/SMC Controllers FR2/Equivalent control/SMC equivalent T2 ==
  theta1ddot : Inport
  theta2 : Inport  Port=2
  theta1 : Inport  Port=3
  theta2ddot : Inport  Port=4
  theta1dot : Inport  Port=5
  Add1 : Sum
  Add2 : Sum
  Add4 : Sum
  Add5 : Sum  Inputs=++++
  Constant : Constant  Value=0.5
  Constant1 : Constant  Value=0.3
  Constant2 : Constant  Value=0.5
  Constant3 : Constant
  Gain10 : Gain  Gain=m2*l2^2
  Gain11 : Gain  Gain=m2*l2
  Gain12 : Gain  Gain=g
  Gain13 : Gain  Gain=(1/3)*(m2*(l2^2))
  Gain5 : Gain  Gain=m2*l1*l2
  Product{1..4,7} (5 alike) : Product
  Product6 : Product  Inputs=3
  Sin : Trigonometry
  Square3 : Math  Operator=square
  Trigonometric Function3 : Trigonometry  Operator=cos
  Trigonometric Function4 : Trigonometry
  T2 : Outport
  wires:
  theta2/1 -> Trigonometric Function3/1, Add4/2, Trigonometric Function4/1
  Trigonometric Function3/1 -> Product3/1
  Gain5/1 -> Product3/2, Product6/1
  Product3/1 -> Add2/1
  Gain10/1 -> Add2/2
  Add2/1 -> Product4/2
  theta1ddot/1 -> Product4/1
  Constant/1 -> Gain5/1
  Constant1/1 -> Gain10/1
  Trigonometric Function4/1 -> Product6/2
  theta1dot/1 -> Square3/1
  Square3/1 -> Product6/3
  Constant2/1 -> Gain11/1
  Gain11/1 -> Gain12/1
  Gain12/1 -> Product7/1
  theta1/1 -> Add4/1
  Sin/1 -> Product7/2
  Add4/1 -> Sin/1
  Product4/1 -> Add5/1
  Product6/1 -> Add5/2
  Product7/1 -> Add5/3
  Add5/1 -> T2/1
  Product1/1 -> Add1/1
  [lamdaBR2] -> Product1/2
  [edotBR2] -> Product1/1
  theta2ddot/1 -> Add1/2
  Constant3/1 -> Gain13/1
  Add1/1 -> Product2/2
  Gain13/1 -> Product2/1
  Product2/1 -> Add5/4

== system singlcontact_control_smc_lqr_mydimes_reaction/Walking Robot/Lqr+Lqr+reaction/SMC Controllers FR3/Equivalent control/SMC equivalent T1 ==
  theta2 : Inport
  theta1 : Inport  Port=2
  theta2ddot : Inport  Port=3
  theta1dot : Inport  Port=4
  theta2dot : Inport  Port=5
  theta1ddot : Inport  Port=6
  Add{1..4} (4 alike) : Sum
  Add5 : Sum  Inputs=+--+++
  Add6 : Sum  Inputs=++++
  Constant : Constant  Value=0.3
  Constant10 : Constant  Value=m2*l1^2
  Constant11 : Constant  Value=0.3*m1*l1^2
  Constant12 : Constant  Value=m2*l1*l2
  Constant2 : Constant  Value=0.5
  Constant3 : Constant
  Constant4 : Constant  Value=0.5
  Constant5 : Constant
  Constant6 : Constant  Value=g*l1
  Constant7 : Constant  Value=0.5
  Constant9 : Constant  Value=0.3*m2*l2^2
  Cos : Trigonometry  Operator=cos
  Cos1 : Trigonometry  Operator=cos
  Gain1 : Gain  Gain=m2*l2^2
  Gain2 : Gain  Gain=m2*l2*l1
  Gain4 : Gain  Gain=m2*l2*l1
  Gain6 : Gain  Gain=m1
  Gain7 : Gain  Gain=m2
  Gain8 : Gain  Gain=m2*g*l2
  Product{1..3,7..9} (6 alike) : Product
  Product4 : Product  Inputs=4
  Product5 : Product  Inputs=3
  Product6 : Product  Inputs=3
  Sin : Trigonometry
  Sin1 : Trigonometry
  Sin2 : Trigonometry
  Square1 : Math  Operator=square
  T1 : Outport
  wires:
  Add2/1 -> Product1/1
  Product9/1 -> Add2/2
  [lamdaBL1] -> Product9/1
  [edotBL1] -> Product9/2
  Add5/1 -> T1/1
  Product1/1 -> Add5/6
  theta1ddot/1 -> Add2/1
  Add6/1 -> Product1/2
  Product8/1 -> Add6/1
  Constant11/1 -> Add6/2
  Constant10/1 -> Add6/4
  Constant9/1 -> Add6/3
  Cos1/1 -> Product8/1
  Constant12/1 -> Product8/2  "X_dd"
  theta2/1 -> Cos/1, Sin/1, Add4/1, Cos1/1
  Product7/1 -> Add5/5
  Product6/1 -> Add5/4
  Product5/1 -> Add5/3
  Product4/1 -> Add5/2
  Product3/1 -> Add5/1
  Sin2/1 -> Product7/2
  Gain8/1 -> Product7/1
  Add4/1 -> Sin2/1
  Constant7/1 -> Gain8/1
  Constant6/1 -> Product6/3
  Sin1/1 -> Product6/2
  Add3/1 -> Product6/1
  theta1/1 -> Sin1/1, Add4/2
  Gain6/1 -> Add3/1
  Gain7/1 -> Add3/2
  Constant5/1 -> Gain7/1
  Constant4/1 -> Gain6/1
  Square1/1 -> Product5/3
  Constant3/1 -> Gain4/1
  Gain4/1 -> Product4/1
  Sin/1 -> Product5/2, Product4/2
  theta2dot/1 -> Square1/1, Product4/4
  theta1dot/1 -> Product4/3
  Add1/1 -> Product3/2
  theta2ddot/1 -> Product3/1
  Product2/1 -> Add1/2
  Gain1/1 -> Add1/1
  Gain2/1 -> Product5/1, Product2/1
  Cos/1 -> Product2/2
  Constant2/1 -> Gain2/1
  Constant/1 -> Gain1/1

== system singlcontact_control_smc_lqr_mydimes_reaction/Walking Robot/Lqr+Lqr+reaction/SMC Controllers FR3/Equivalent control/SMC equivalent T2 ==
  theta1ddot : Inport
  theta2 : Inport  Port=2
  theta1 : Inport  Port=3
  theta2ddot : Inport  Port=4
  theta1dot : Inport  Port=5
  Add1 : Sum
  Add2 : Sum
  Add4 : Sum
  Add5 : Sum  Inputs=++++
  Constant : Constant  Value=0.5
  Constant1 : Constant  Value=0.3
  Constant2 : Constant  Value=0.5
  Constant3 : Constant
  Gain10 : Gain  Gain=m2*l2^2
  Gain11 : Gain  Gain=m2*l2
  Gain12 : Gain  Gain=g
  Gain13 : Gain  Gain=(1/3)*(m2*(l2^2))
  Gain5 : Gain  Gain=m2*l1*l2
  Product{1..4,7} (5 alike) : Product
  Product6 : Product  Inputs=3
  Sin : Trigonometry
  Square3 : Math  Operator=square
  Trigonometric Function3 : Trigonometry  Operator=cos
  Trigonometric Function4 : Trigonometry
  T2 : Outport
  wires:
  Product2/1 -> Add5/4
  Gain13/1 -> Product2/1
  Add1/1 -> Product2/2
  Constant3/1 -> Gain13/1
  theta2ddot/1 -> Add1/2
  [edotBL2] -> Product1/1
  [lamdaBL2] -> Product1/2
  Product1/1 -> Add1/1
  Add5/1 -> T2/1
  Product7/1 -> Add5/3
  Product6/1 -> Add5/2
  Product4/1 -> Add5/1
  Add4/1 -> Sin/1
  Sin/1 -> Product7/2
  theta1/1 -> Add4/1
  Gain12/1 -> Product7/1
  Gain11/1 -> Gain12/1
  Constant2/1 -> Gain11/1
  Square3/1 -> Product6/3
  theta1dot/1 -> Square3/1
  Trigonometric Function4/1 -> Product6/2
  Constant1/1 -> Gain10/1
  Constant/1 -> Gain5/1
  theta1ddot/1 -> Product4/1
  Add2/1 -> Product4/2
  Gain10/1 -> Add2/2
  Product3/1 -> Add2/1
  Gain5/1 -> Product6/1, Product3/2
  Trigonometric Function3/1 -> Product3/1
  theta2/1 -> Trigonometric Function4/1, Add4/2, Trigonometric Function3/1

== system singlcontact_control_smc_lqr_mydimes_reaction/Walking Robot/Pid+Pid+reaction1/PID Controllers FR4/Subsystem2/length from ground ==
  In1 : Inport
  In2 : Inport  Port=2
  Gain1 : Gain  Gain=l1
  Gain3 : Gain  Gain=l1
  Gain4 : Gain  Gain=l2
  Sin : Trigonometry
  Sin1 : Trigonometry
  Sin3 : Trigonometry
  Sum : Sum  Inputs=|++
  Sum2 : Sum  Inputs=|++
  Output : Outport
  Outport : Outport  Port=2
  wires:
  In1/1 -> Sin/1, Sum2/1, Sin1/1
  Sin/1 -> Gain1/1
  Gain4/1 -> Sum/2
  Gain3/1 -> Sum/1
  Sum2/1 -> Sin3/1
  Sin1/1 -> Gain3/1
  Sin3/1 -> Gain4/1
  In2/1 -> Sum2/2
  Gain1/1 -> Output/1
  Sum/1 -> Outport/1

== system singlcontact_control_smc_lqr_mydimes_reaction/Walking Robot/Pid+Pid+reaction1/PID Controllers FR5/Subsystem2/length from ground ==
  In1 : Inport
  In2 : Inport  Port=2
  Gain1 : Gain  Gain=l1
  Gain3 : Gain  Gain=l1
  Gain4 : Gain  Gain=l2
  Sin : Trigonometry
  Sin1 : Trigonometry
  Sin3 : Trigonometry
  Sum : Sum  Inputs=|++
  Sum2 : Sum  Inputs=|++
  Output : Outport
  Outport : Outport  Port=2
  wires:
  In1/1 -> Sin/1, Sum2/1, Sin1/1
  Sin/1 -> Gain1/1
  Gain4/1 -> Sum/2
  Gain3/1 -> Sum/1
  Sum2/1 -> Sin3/1
  Sin1/1 -> Gain3/1
  Sin3/1 -> Gain4/1
  In2/1 -> Sum2/2
  Gain1/1 -> Output/1
  Sum/1 -> Outport/1

== system singlcontact_control_smc_lqr_mydimes_reaction/Walking Robot/Pid+Pid+reaction1/PID Controllers FR6/Subsystem2/length from ground ==
  In1 : Inport
  In2 : Inport  Port=2
  Gain1 : Gain  Gain=l1
  Gain3 : Gain  Gain=l1
  Gain4 : Gain  Gain=l2
  Sin : Trigonometry
  Sin1 : Trigonometry
  Sin3 : Trigonometry
  Sum : Sum  Inputs=|++
  Sum2 : Sum  Inputs=|++
  Output : Outport
  Outport : Outport  Port=2
  wires:
  In1/1 -> Sin/1, Sum2/1, Sin1/1
  Sin/1 -> Gain1/1
  Gain4/1 -> Sum/2
  Gain3/1 -> Sum/1
  Sum2/1 -> Sin3/1
  Sin1/1 -> Gain3/1
  Sin3/1 -> Gain4/1
  In2/1 -> Sum2/2
  Gain1/1 -> Output/1
  Sum/1 -> Outport/1

== system singlcontact_control_smc_lqr_mydimes_reaction/Walking Robot/Pid+Pid+reaction1/PID Controllers FR7/Subsystem2/length from ground ==
  In1 : Inport
  In2 : Inport  Port=2
  Gain1 : Gain  Gain=l1
  Gain3 : Gain  Gain=l1
  Gain4 : Gain  Gain=l2
  Sin : Trigonometry
  Sin1 : Trigonometry
  Sin3 : Trigonometry
  Sum : Sum  Inputs=|++
  Sum2 : Sum  Inputs=|++
  Output : Outport
  Outport : Outport  Port=2
  wires:
  In1/1 -> Sin/1, Sum2/1, Sin1/1
  Sin/1 -> Gain1/1
  Gain4/1 -> Sum/2
  Gain3/1 -> Sum/1
  Sum2/1 -> Sin3/1
  Sin1/1 -> Gain3/1
  Sin3/1 -> Gain4/1
  In2/1 -> Sum2/2
  Gain1/1 -> Output/1
  Sum/1 -> Outport/1

== system singlcontact_control_smc_lqr_mydimes_reaction/Walking Robot/Pid+Pid+reaction1/SMC Controllers FR1/Equivalent control/SMC equivalent T1 ==
  theta2 : Inport
  theta1 : Inport  Port=2
  theta2ddot : Inport  Port=3
  theta1dot : Inport  Port=4
  theta2dot : Inport  Port=5
  theta1ddot : Inport  Port=6
  Add{1..4} (4 alike) : Sum
  Add5 : Sum  Inputs=+--+++
  Add6 : Sum  Inputs=++++
  Constant : Constant  Value=0.3
  Constant10 : Constant  Value=m2*l1^2
  Constant11 : Constant  Value=0.3*m1*l1^2
  Constant12 : Constant  Value=m2*l1*l2
  Constant2 : Constant  Value=0.5
  Constant3 : Constant
  Constant4 : Constant  Value=0.5
  Constant5 : Constant
  Constant6 : Constant  Value=g*l1
  Constant7 : Constant  Value=0.5
  Constant9 : Constant  Value=0.3*m2*l2^2
  Cos : Trigonometry  Operator=cos
  Cos1 : Trigonometry  Operator=cos
  Gain1 : Gain  Gain=m2*l2^2
  Gain2 : Gain  Gain=m2*l2*l1
  Gain4 : Gain  Gain=m2*l2*l1
  Gain6 : Gain  Gain=m1
  Gain7 : Gain  Gain=m2
  Gain8 : Gain  Gain=m2*g*l2
  Product{1..3,7..9} (6 alike) : Product
  Product4 : Product  Inputs=4
  Product5 : Product  Inputs=3
  Product6 : Product  Inputs=3
  Sin : Trigonometry
  Sin1 : Trigonometry
  Sin2 : Trigonometry
  Square1 : Math  Operator=square
  T1 : Outport
  wires:
  Add2/1 -> Product1/1
  Product9/1 -> Add2/2
  [lamdaFL1] -> Product9/1
  [edotFL1] -> Product9/2
  Add5/1 -> T1/1
  Product1/1 -> Add5/6
  theta1ddot/1 -> Add2/1
  Add6/1 -> Product1/2
  Product8/1 -> Add6/1
  Constant11/1 -> Add6/2
  Constant10/1 -> Add6/4
  Constant9/1 -> Add6/3
  Cos1/1 -> Product8/1
  Constant12/1 -> Product8/2  "X_dd"
  theta2/1 -> Cos/1, Sin/1, Add4/1, Cos1/1
  Product7/1 -> Add5/5
  Product6/1 -> Add5/4
  Product5/1 -> Add5/3
  Product4/1 -> Add5/2
  Product3/1 -> Add5/1
  Sin2/1 -> Product7/2
  Gain8/1 -> Product7/1
  Add4/1 -> Sin2/1
  Constant7/1 -> Gain8/1
  Constant6/1 -> Product6/3
  Sin1/1 -> Product6/2
  Add3/1 -> Product6/1
  theta1/1 -> Sin1/1, Add4/2
  Gain6/1 -> Add3/1
  Gain7/1 -> Add3/2
  Constant5/1 -> Gain7/1
  Constant4/1 -> Gain6/1
  Square1/1 -> Product5/3
  Constant3/1 -> Gain4/1
  Gain4/1 -> Product4/1
  Sin/1 -> Product5/2, Product4/2
  theta2dot/1 -> Square1/1, Product4/4
  theta1dot/1 -> Product4/3
  Add1/1 -> Product3/2
  theta2ddot/1 -> Product3/1
  Product2/1 -> Add1/2
  Gain1/1 -> Add1/1
  Gain2/1 -> Product5/1, Product2/1
  Cos/1 -> Product2/2
  Constant2/1 -> Gain2/1
  Constant/1 -> Gain1/1

== system singlcontact_control_smc_lqr_mydimes_reaction/Walking Robot/Pid+Pid+reaction1/SMC Controllers FR1/Equivalent control/SMC equivalent T2 ==
  theta1ddot : Inport
  theta2 : Inport  Port=2
  theta1 : Inport  Port=3
  theta2ddot : Inport  Port=4
  theta1dot : Inport  Port=5
  Add1 : Sum
  Add2 : Sum
  Add4 : Sum
  Add5 : Sum  Inputs=++++
  Constant : Constant  Value=0.5
  Constant1 : Constant  Value=0.3
  Constant2 : Constant  Value=0.5
  Constant3 : Constant
  Gain10 : Gain  Gain=m2*l2^2
  Gain11 : Gain  Gain=m2*l2
  Gain12 : Gain  Gain=g
  Gain13 : Gain  Gain=(1/3)*(m2*(l2^2))
  Gain5 : Gain  Gain=m2*l1*l2
  Product{1..4,7} (5 alike) : Product
  Product6 : Product  Inputs=3
  Sin : Trigonometry
  Square3 : Math  Operator=square
  Trigonometric Function3 : Trigonometry  Operator=cos
  Trigonometric Function4 : Trigonometry
  T2 : Outport
  wires:
  Product2/1 -> Add5/4
  Gain13/1 -> Product2/1
  Add1/1 -> Product2/2
  Constant3/1 -> Gain13/1
  theta2ddot/1 -> Add1/2
  [edotFL2] -> Product1/1
  [lamdaFL2] -> Product1/2
  Product1/1 -> Add1/1
  Add5/1 -> T2/1
  Product7/1 -> Add5/3
  Product6/1 -> Add5/2
  Product4/1 -> Add5/1
  Add4/1 -> Sin/1
  Sin/1 -> Product7/2
  theta1/1 -> Add4/1
  Gain12/1 -> Product7/1
  Gain11/1 -> Gain12/1
  Constant2/1 -> Gain11/1
  Square3/1 -> Product6/3
  theta1dot/1 -> Square3/1
  Trigonometric Function4/1 -> Product6/2
  Constant1/1 -> Gain10/1
  Constant/1 -> Gain5/1
  theta1ddot/1 -> Product4/1
  Add2/1 -> Product4/2
  Gain10/1 -> Add2/2
  Product3/1 -> Add2/1
  Gain5/1 -> Product6/1, Product3/2
  Trigonometric Function3/1 -> Product3/1
  theta2/1 -> Trigonometric Function4/1, Add4/2, Trigonometric Function3/1

== system singlcontact_control_smc_lqr_mydimes_reaction/Walking Robot/Pid+Pid+reaction1/SMC Controllers FR2/Equivalent control/SMC equivalent T1 ==
  theta2 : Inport
  theta1 : Inport  Port=2
  theta2ddot : Inport  Port=3
  theta1dot : Inport  Port=4
  theta2dot : Inport  Port=5
  theta1ddot : Inport  Port=6
  Add{1..4} (4 alike) : Sum
  Add5 : Sum  Inputs=+--+++
  Add6 : Sum  Inputs=++++
  Constant : Constant  Value=0.3
  Constant10 : Constant  Value=m2*l1^2
  Constant11 : Constant  Value=0.3*m1*l1^2
  Constant12 : Constant  Value=m2*l1*l2
  Constant2 : Constant  Value=0.5
  Constant3 : Constant
  Constant4 : Constant  Value=0.5
  Constant5 : Constant
  Constant6 : Constant  Value=g*l1
  Constant7 : Constant  Value=0.5
  Constant9 : Constant  Value=0.3*m2*l2^2
  Cos : Trigonometry  Operator=cos
  Cos1 : Trigonometry  Operator=cos
  Gain1 : Gain  Gain=m2*l2^2
  Gain2 : Gain  Gain=m2*l2*l1
  Gain4 : Gain  Gain=m2*l2*l1
  Gain6 : Gain  Gain=m1
  Gain7 : Gain  Gain=m2
  Gain8 : Gain  Gain=m2*g*l2
  Product{1..3,7..9} (6 alike) : Product
  Product4 : Product  Inputs=4
  Product5 : Product  Inputs=3
  Product6 : Product  Inputs=3
  Sin : Trigonometry
  Sin1 : Trigonometry
  Sin2 : Trigonometry
  Square1 : Math  Operator=square
  T1 : Outport
  wires:
  Constant/1 -> Gain1/1
  Constant2/1 -> Gain2/1
  Cos/1 -> Product2/2
  Gain2/1 -> Product2/1, Product5/1
  Gain1/1 -> Add1/1
  Product2/1 -> Add1/2
  theta2ddot/1 -> Product3/1
  Add1/1 -> Product3/2
  theta1dot/1 -> Product4/3
  theta2dot/1 -> Product4/4, Square1/1
  Sin/1 -> Product4/2, Product5/2
  Gain4/1 -> Product4/1
  Constant3/1 -> Gain4/1
  Square1/1 -> Product5/3
  Constant4/1 -> Gain6/1
  Constant5/1 -> Gain7/1
  Gain7/1 -> Add3/2
  Gain6/1 -> Add3/1
  theta1/1 -> Add4/2, Sin1/1
  Add3/1 -> Product6/1
  Sin1/1 -> Product6/2
  Constant6/1 -> Product6/3
  Constant7/1 -> Gain8/1
  Add4/1 -> Sin2/1
  Gain8/1 -> Product7/1
  Sin2/1 -> Product7/2
  Product3/1 -> Add5/1
  Product4/1 -> Add5/2
  Product5/1 -> Add5/3
  Product6/1 -> Add5/4
  Product7/1 -> Add5/5
  theta2/1 -> Cos1/1, Add4/1, Sin/1, Cos/1
  Constant12/1 -> Product8/2  "X_dd"
  Cos1/1 -> Product8/1
  Constant9/1 -> Add6/3
  Constant10/1 -> Add6/4
  Constant11/1 -> Add6/2
  Product8/1 -> Add6/1
  Add6/1 -> Product1/2
  theta1ddot/1 -> Add2/1
  Product1/1 -> Add5/6
  Add5/1 -> T1/1
  [edotBR1] -> Product9/2
  [lamdaBR1] -> Product9/1
  Product9/1 -> Add2/2
  Add2/1 -> Product1/1

== system singlcontact_control_smc_lqr_mydimes_reaction/Walking Robot/Pid+Pid+reaction1/SMC Controllers FR2/Equivalent control/SMC equivalent T2 ==
  theta1ddot : Inport
  theta2 : Inport  Port=2
  theta1 : Inport  Port=3
  theta2ddot : Inport  Port=4
  theta1dot : Inport  Port=5
  Add1 : Sum
  Add2 : Sum
  Add4 : Sum
  Add5 : Sum  Inputs=++++
  Constant : Constant  Value=0.5
  Constant1 : Constant  Value=0.3
  Constant2 : Constant  Value=0.5
  Constant3 : Constant
  Gain10 : Gain  Gain=m2*l2^2
  Gain11 : Gain  Gain=m2*l2
  Gain12 : Gain  Gain=g
  Gain13 : Gain  Gain=(1/3)*(m2*(l2^2))
  Gain5 : Gain  Gain=m2*l1*l2
  Product{1..4,7} (5 alike) : Product
  Product6 : Product  Inputs=3
  Sin : Trigonometry
  Square3 : Math  Operator=square
  Trigonometric Function3 : Trigonometry  Operator=cos
  Trigonometric Function4 : Trigonometry
  T2 : Outport
  wires:
  theta2/1 -> Trigonometric Function3/1, Add4/2, Trigonometric Function4/1
  Trigonometric Function3/1 -> Product3/1
  Gain5/1 -> Product3/2, Product6/1
  Product3/1 -> Add2/1
  Gain10/1 -> Add2/2
  Add2/1 -> Product4/2
  theta1ddot/1 -> Product4/1
  Constant/1 -> Gain5/1
  Constant1/1 -> Gain10/1
  Trigonometric Function4/1 -> Product6/2
  theta1dot/1 -> Square3/1
  Square3/1 -> Product6/3
  Constant2/1 -> Gain11/1
  Gain11/1 -> Gain12/1
  Gain12/1 -> Product7/1
  theta1/1 -> Add4/1
  Sin/1 -> Product7/2
  Add4/1 -> Sin/1
  Product4/1 -> Add5/1
  Product6/1 -> Add5/2
  Product7/1 -> Add5/3
  Add5/1 -> T2/1
  Product1/1 -> Add1/1
  [lamdaBR2] -> Product1/2
  [edotBR2] -> Product1/1
  theta2ddot/1 -> Add1/2
  Constant3/1 -> Gain13/1
  Add1/1 -> Product2/2
  Gain13/1 -> Product2/1
  Product2/1 -> Add5/4
